simulink model "Simulink_sistema"  (R2023b)
settings: Solver=VariableStepAuto  StartTime=0.0  StopTime=5  RelTol=1e-3
undefined symbols (not defined in the file): k, m, r
settings Model: Creator=USER  LastModifiedBy=USER

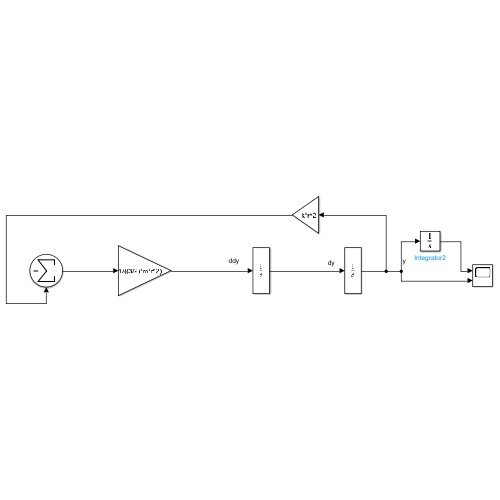
[thumbnail: Simulink's stored preview of the top-level diagram]
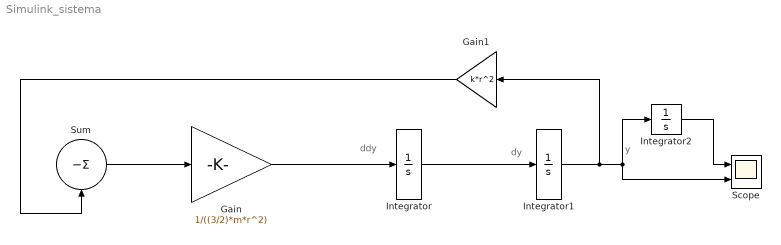
== system Simulink_sistema ==
  note: y
  note: ddy
  note: dy
  Gain : Gain  Gain=1/((3/2)*m*r^2)
  Gain1 : Gain  Gain=k*r^2
  Integrator : Integrator
  Integrator1 : Integrator  InitialCondition=2
  Integrator2 : Integrator
  Scope : Scope  NumInputPorts=2
  Sum : Sum  Inputs=|-
  wires:
  Gain/1 -> Integrator/1
  Sum/1 -> Gain/1
  Integrator/1 -> Integrator1/1
  Integrator1/1 -> Gain1/1, Scope/2, Integrator2/1
  Gain1/1 -> Sum/1
  Integrator2/1 -> Scope/1
